simulink model "untitled"  (R2013a)
settings: Solver=ode45  StartTime=0.0  StopTime=10.0  RelTol=1e-3
undefined symbols (not defined in the file): fdesignblkfcn, gcbh
libraries: simulink x2
settings Model: Creator=user  LastModifiedBy=user

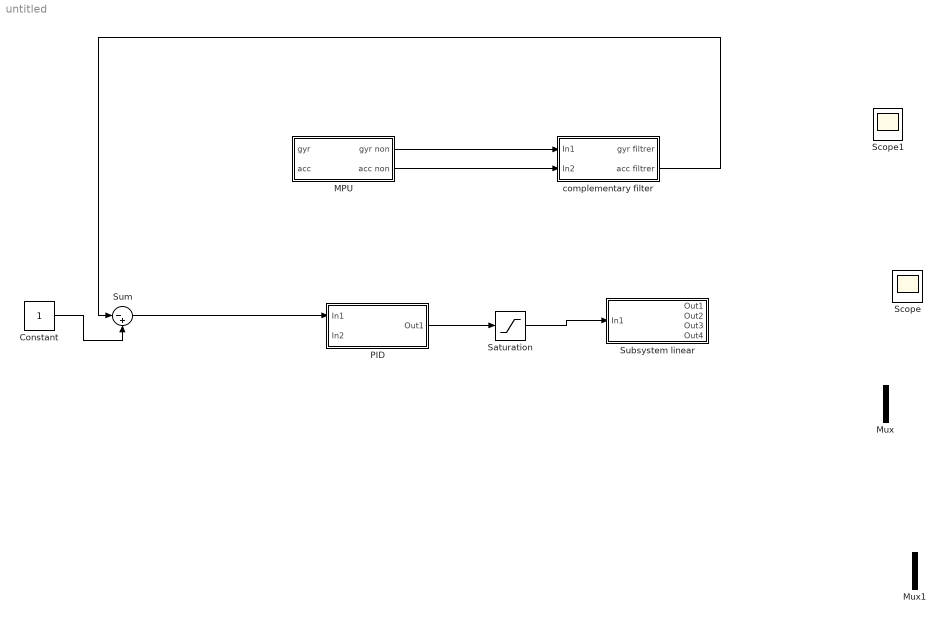
== system untitled ==
  Constant : Constant
  "MPU " : Subsystem
  Mux : Mux  Inputs=2
  Mux1 : Mux  Inputs=2
  PID : Subsystem
  Saturation : Saturate
  Scope : Scope
  Scope1 : Scope
  Subsystem linear : Subsystem
  Sum : Sum  Inputs=|-+
  complementary filter : Subsystem
  wires:
  Constant/1 -> Sum/2
  complementary filter/2(acc filtrer) -> Sum/1
  Sum/1 -> PID/1(In1)
  PID/1(Out1) -> Saturation/1
  Saturation/1 -> Subsystem linear/1(In1)
  "MPU "/1(gyr non) -> complementary filter/1(In1)
  "MPU "/2("acc non ") -> complementary filter/2(In2)

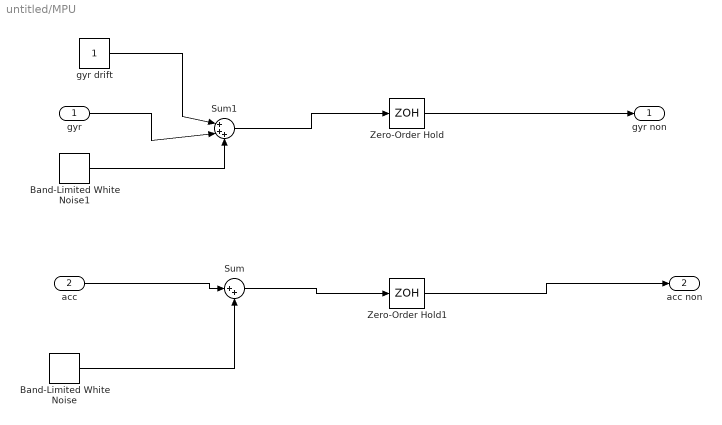
== system untitled/MPU  ==
  gyr : Inport
  acc : Inport  Port=2
  Band-Limited White Noise : simulink/Sources/Band-Limited White Noise  Cov=[0.1]  Ts=0.1  seed=[23341]
  Band-Limited White Noise1 : simulink/Sources/Band-Limited White Noise  Cov=[0.1]  Ts=0.1  seed=[23341]
  Sum : Sum  Inputs=|++
  Sum1 : Sum  Inputs=|+++
  Zero-Order Hold : ZeroOrderHold
  Zero-Order Hold1 : ZeroOrderHold
  gyr drift : Constant
  gyr non : Outport
  "acc non " : Outport  Port=2
  wires:
  gyr/1 -> Sum1/2
  acc/1 -> Sum/1
  Band-Limited White Noise1/1 -> Sum1/3
  Band-Limited White Noise/1 -> Sum/2
  gyr drift/1 -> Sum1/1
  Sum1/1 -> Zero-Order Hold/1
  Sum/1 -> Zero-Order Hold1/1
  Zero-Order Hold1/1 -> "acc non "/1
  Zero-Order Hold/1 -> gyr non/1

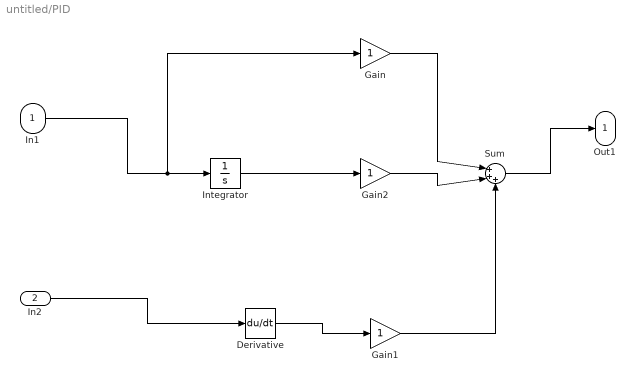
== system untitled/PID ==
  In1 : Inport  PortDimensions=1  SampleTime=2  LockScale=on
  In2 : Inport  Port=2
  Derivative : Derivative
  Gain : Gain
  Gain1 : Gain
  Gain2 : Gain
  Integrator : Integrator
  Sum : Sum  Inputs=|+++
  Out1 : Outport
  wires:
  Integrator/1 -> Gain2/1
  Gain/1 -> Sum/1
  Gain2/1 -> Sum/2
  Gain1/1 -> Sum/3
  Sum/1 -> Out1/1
  In1/1 -> Gain/1, Integrator/1
  Derivative/1 -> Gain1/1
  In2/1 -> Derivative/1

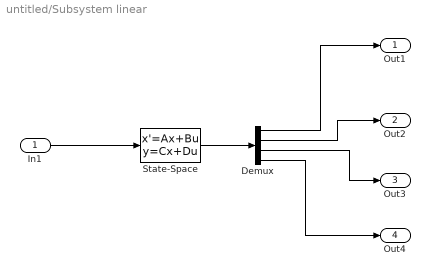
== system untitled/Subsystem linear ==
  In1 : Inport
  Demux : Demux
  State-Space : StateSpace
  Out1 : Outport
  Out2 : Outport  Port=2
  Out3 : Outport  Port=3
  Out4 : Outport  Port=4
  wires:
  Demux/1 -> Out1/1
  Demux/2 -> Out2/1
  Demux/3 -> Out3/1
  Demux/4 -> Out4/1
  State-Space/1 -> Demux/1
  In1/1 -> State-Space/1

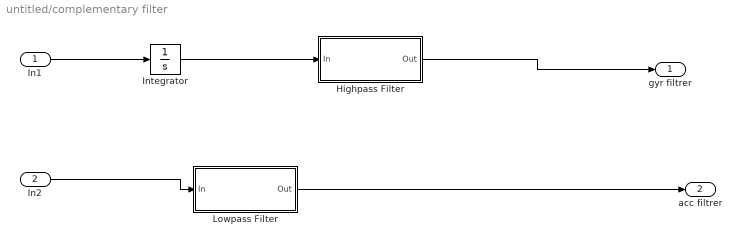
== system untitled/complementary filter ==
  In1 : Inport
  In2 : Inport  Port=2
  Highpass Filter : Subsystem  DialogController=fdesignblkfcn  InitFcn=fdesignblkfcn(gcbh, {'InitFcn'});  mask(Highpass Filter){}
      mask help: Design a highpass filter
      settings: CopyFcn=fdesignblkfcn(gcbh, {'CopyFcn'});
      mask Help: helpview(mapfilelocation('dsp'), 'dsphighpassfilter');
      mask Display: disp('Highpass')
  Integrator : Integrator
  Lowpass Filter : Subsystem  DialogController=fdesignblkfcn  InitFcn=fdesignblkfcn(gcbh, {'InitFcn'});  mask(Lowpass Filter){}
      mask help: Design a lowpass filter
      settings: CopyFcn=fdesignblkfcn(gcbh, {'CopyFcn'});
      mask Help: helpview(mapfilelocation('dsp'), 'dsplowpassfilter');
      mask Display: disp('Lowpass')
  gyr filtrer : Outport
  acc filtrer : Outport  Port=2
  wires:
  In2/1 -> Lowpass Filter/1(In)
  In1/1 -> Integrator/1
  Integrator/1 -> Highpass Filter/1(In)
  Highpass Filter/1(Out) -> gyr filtrer/1
  Lowpass Filter/1(Out) -> acc filtrer/1

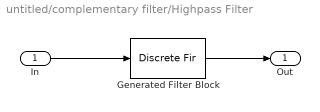
== system untitled/complementary filter/Highpass Filter ==
  In : Inport
  Generated Filter Block : DiscreteFir  Tag=BlockMethodSubSystem  Coefficients=[-0.001713682665110306 0.0083143784480805769 -0.012717355233486931 0.0055609517902503753 0.0073397102425536197 -0.006531049050179258 -0.0076900499697794954 0.0090269831680985079 0.0088388618995090904 -0.012960741353766195 -0.010074958667252783 0.018520174010008873 0.011233354613588929 -0.026375248383613631 -0.012270782185765867 0.038180976692389727 0.013130425918293593 -0.058293359325192265 -0.013768295948648092 0.102813257992074 0.014167876773854067 -0.31720255241603534 0.48569804617051759 -0.31720255241603534 0.014167876773854067 0.102813257992074 -0.013768295948648092 -0.058293359325192265 0.013130425918293593 0.038180976692389727 -0.012270782185765867 -0.026375248383613631 0.011233354613588929 0.018520174010008873 -0.010074958667252783 -0.012960741353766195 0.0088388618995090904 0.0090269831680985079 -0.0076900499697794954 -0.006531049050179258 0.0073397102425536197 0.0055609517902503753 -0.012717355233486931 0.0083143784480805769 -0.001713682665110306]  InputProcessing=Columns as channels (frame based)
  Out : Outport
  wires:
  Generated Filter Block/1 -> Out/1
  In/1 -> Generated Filter Block/1

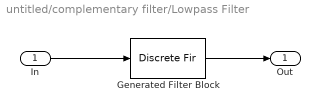
== system untitled/complementary filter/Lowpass Filter ==
  In : Inport
  Generated Filter Block : DiscreteFir  Tag=BlockMethodSubSystem  Coefficients=[-0.0024228738523269142 -0.002083244982079274 0.0067703446401187091 0.016731945423489058 0.011117076081077608 -0.0062311454141445394 -0.008401617186026911 0.0092567976151380175 0.012982883808855752 -0.010121234703278968 -0.018273518733782485 0.011431962071777957 0.02617588858040763 -0.012489027835322923 -0.037996623145463579 0.013388945199366963 0.058155465814729891 -0.014048043515808939 -0.10272466857882172 0.014462275771238358 0.31716649721769491 0.48538764678732504 0.31716649721769491 0.014462275771238358 -0.10272466857882172 -0.014048043515808939 0.058155465814729891 0.013388945199366963 -0.037996623145463579 -0.012489027835322923 0.02617588858040763 0.011431962071777957 -0.018273518733782485 -0.010121234703278968 0.012982883808855752 0.0092567976151380175 -0.008401617186026911 -0.0062311454141445394 0.011117076081077608 0.016731945423489058 0.0067703446401187091 -0.002083244982079274 -0.0024228738523269142]  InputProcessing=Columns as channels (frame based)
  Out : Outport
  wires:
  In/1 -> Generated Filter Block/1
  Generated Filter Block/1 -> Out/1
